simulink model "M9_sim"  (R2021b)
settings: Solver=VariableStepAuto  StartTime=0.0  StopTime=10.0  RelTol=1e-3
values from neighbouring files (symbols this model uses):
  K1 = wn^2    [M12.m]    (also in M9.m)
  K2 = (2*zeta*wn + K1) / K1    [M12.m]    (also in M9.m = (2*zeta*wn + 1) / K1)
  wn = wr/sqrt(1-2*zeta^2)    [M12.m]    (also in M9.m = (1+0.7*zeta) / to)
  zeta = rzeta(4)    [M12.m]    (also in M9.m)
settings Model: Creator=Studenci  LastModifiedBy=Studenci

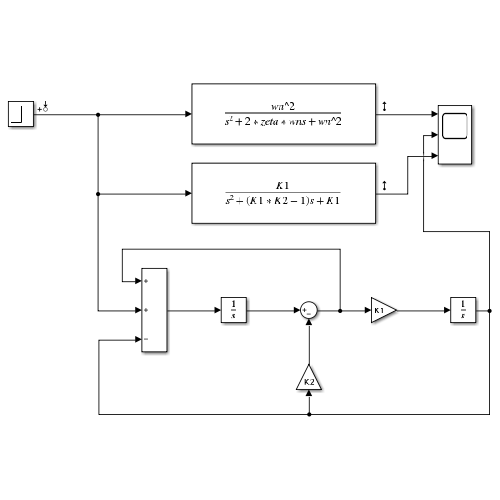
[thumbnail: Simulink's stored preview of the top-level diagram]
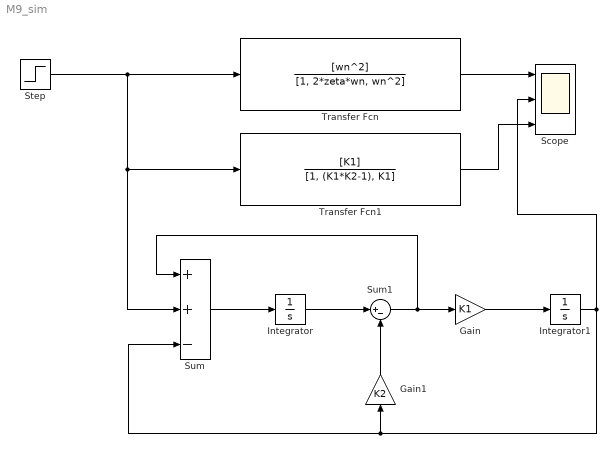
== system M9_sim ==
  Gain : Gain  Gain=K1
  Gain1 : Gain  Gain=K2
  Integrator : Integrator
  Integrator1 : Integrator
  Scope : Scope  NumInputPorts=3
  Step : Step  Time=0  SampleTime=0
  Sum : Sum  Inputs=++-
  Sum1 : Sum  Inputs=|+-
  Transfer Fcn : TransferFcn  Numerator=[wn^2]  Denominator=[1, 2*zeta*wn, wn^2]
  Transfer Fcn1 : TransferFcn  Numerator=[K1]  Denominator=[1, (K1*K2-1), K1]
  wires:
  Step/1 -> Sum/2, Transfer Fcn1/1, Transfer Fcn/1
  Transfer Fcn/1 -> Scope/1
  Sum/1 -> Integrator/1
  Integrator/1 -> Sum1/1
  Sum1/1 -> Sum/1, Gain/1
  Gain1/1 -> Sum1/2
  Gain/1 -> Integrator1/1
  Integrator1/1 -> Scope/2, Sum/3, Gain1/1
  Transfer Fcn1/1 -> Scope/3
